simulink model "three_phase_bidirectional_EV_charger_simscape"  (R2019a)
settings: Solver=ode23tb  StartTime=0.0  StopTime=0.2  MaxStep=1e-5  RelTol=1e-5
values from neighbouring files (symbols this model uses):
  C = 33e-6    (= 3.3e-05)    [parameters_for_g2v_closed_loop.m]    (also in parameters_for_v2g_closed_loop.m = 0.002)
  Cf = 300e-3    (= 0.3)    [parameters_for_g2v_closed_loop.m]    (also in parameters_for_v2g_closed_loop.m)
  Co = 2e-3    (= 0.002)    [parameters_for_g2v_closed_loop.m]    (also in parameters_for_v2g_closed_loop.m)
  fline = 50    [parameters_for_g2v_closed_loop.m]    (also in parameters_for_v2g_closed_loop.m)
  fsw_dc = 100e3    (= 100000)    [parameters_for_g2v_closed_loop.m]    (also in parameters_for_v2g_closed_loop.m)
  H = 0.0075    [parameters_for_g2v_closed_loop.m]    (also in parameters_for_v2g_closed_loop.m)
  I = V/R    (= 10)    [parameters_for_g2v_closed_loop.m]    (also in parameters_for_v2g_closed_loop.m = V/(R*(1-D)))
  indicator = 1    [parameters_for_g2v_closed_loop.m]    (also in parameters_for_v2g_closed_loop.m = 0)
  Iqe_max = -Idc_max/K    (= -16.4102564103)    [parameters_for_g2v_closed_loop.m]    (also in parameters_for_v2g_closed_loop.m)
  Kic = Kpc/Tc    (= 4545.45454545)    [parameters_for_g2v_closed_loop.m]    (also in parameters_for_v2g_closed_loop.m)
  Kic_dc = 6749.8    [parameters_for_g2v_closed_loop.m]    (also in parameters_for_v2g_closed_loop.m = 9270.6)
  Kipll = Kpll/Tpll    [parameters_for_g2v_closed_loop.m]    (also in parameters_for_v2g_closed_loop.m)
  Kiv = Kpv/Tv_ac    [parameters_for_g2v_closed_loop.m]    (also in parameters_for_v2g_closed_loop.m)
  Kiv_dc = 15687    [parameters_for_g2v_closed_loop.m]    (also in parameters_for_v2g_closed_loop.m = 1260000)
  Kpc = Kc    (= 32.7272727273)    [parameters_for_g2v_closed_loop.m]    (also in parameters_for_v2g_closed_loop.m)
  Kpc_dc = 0.3    [parameters_for_g2v_closed_loop.m]    (also in parameters_for_v2g_closed_loop.m = 0.29)
  Kpll = (1/Vm)*(1/(alfa_pll*Tsamp_ac))    [parameters_for_g2v_closed_loop.m]    (also in parameters_for_v2g_closed_loop.m)
  Kpv = Kv    [parameters_for_g2v_closed_loop.m]    (also in parameters_for_v2g_closed_loop.m)
  Kpv_dc = 6.9    [parameters_for_g2v_closed_loop.m]    (also in parameters_for_v2g_closed_loop.m = 625.3)
  L = 250e-6    (= 0.00025)    [parameters_for_g2v_closed_loop.m]    (also in parameters_for_v2g_closed_loop.m)
  Lg = 1e-3    (= 0.001)    [parameters_for_g2v_closed_loop.m]    (also in parameters_for_v2g_closed_loop.m)
  Li = 1.6e-3    (= 0.0016)    [parameters_for_g2v_closed_loop.m]    (also in parameters_for_v2g_closed_loop.m)
  Ls = 1e-3    (= 0.001)    [parameters_for_g2v_closed_loop.m]    (also in parameters_for_v2g_closed_loop.m)
  R = V/Iload    (= 50)    [parameters_for_g2v_closed_loop.m]    (also in parameters_for_v2g_closed_loop.m = 1000000)
  Resr = 6e-3    (= 0.006)    [parameters_for_g2v_closed_loop.m]    (also in parameters_for_v2g_closed_loop.m = 0)
  Rf = 0.25    [parameters_for_g2v_closed_loop.m]    (also in parameters_for_v2g_closed_loop.m)
  RL = 10e-3    (= 0.01)    [parameters_for_g2v_closed_loop.m]    (also in parameters_for_v2g_closed_loop.m)
  Rs = 0.5    [parameters_for_g2v_closed_loop.m]    (also in parameters_for_v2g_closed_loop.m)
  T1 = Tsamp_ac/10    (= 5e-06)    [parameters_for_g2v_closed_loop.m]    (also in parameters_for_v2g_closed_loop.m)
  T2 = Tsamp_ac/10    (= 5e-06)    [parameters_for_g2v_closed_loop.m]    (also in parameters_for_v2g_closed_loop.m)
  Tsamp_ac = Tsw_ac/2    (= 5e-05)    [parameters_for_g2v_closed_loop.m]    (also in parameters_for_v2g_closed_loop.m)
  Tsamp_dc = Tsw_dc/2    (= 5e-06)    [parameters_for_g2v_closed_loop.m]    (also in parameters_for_v2g_closed_loop.m)
  V = 500    [parameters_for_g2v_closed_loop.m]    (also in parameters_for_v2g_closed_loop.m = 800)
  Vdc = 800    [parameters_for_g2v_closed_loop.m]    (also in parameters_for_v2g_closed_loop.m)
  Vm = 325    [parameters_for_g2v_closed_loop.m]    (also in parameters_for_v2g_closed_loop.m)
  VM = 4    [parameters_for_g2v_closed_loop.m]    (also in parameters_for_v2g_closed_loop.m)
undefined symbols (not defined in the file or in its folder): Ion, Lithium
libraries: powerlib x58, simulink x9, powerlib_meascontrol x1, electricdrivelib x1
(part 1 of 2)
settings Model: Creator=Görkem  LastModifiedBy=gsahi
settings DataIOCC: ReturnWorkspaceOutputs=off
settings DebuggingCC: ParameterOverflowMsg=none
settings SimscapeCC: SimscapeLogType=all

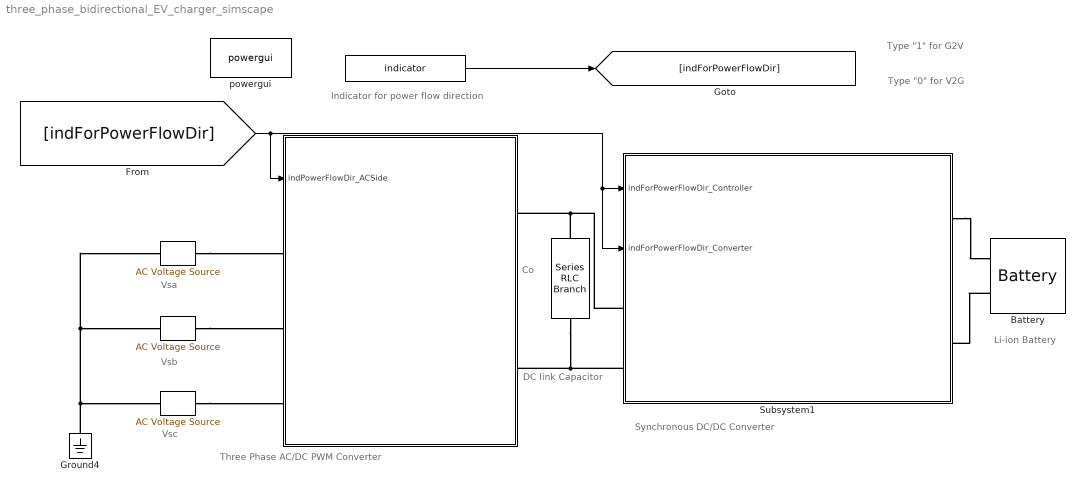
== system three_phase_bidirectional_EV_charger_simscape ==
  note: Vsa
  note: DC link
      | Capacitor
  note: Synchronous DC/DC Converter
  note: Three Phase AC/DC PWM Converter
  note: Indicator for power flow direction
  note: Type "1" for G2V
  note: Type "0" for V2G
  note: Vsb
  note: Vsc
  note: Li-ion
      | Battery
  note: Co
  " " : powerlib/Elements/Series RLC Branch  LConnTagsString=__new0  RConnTagsString=__new0  BranchType=C  Resistance=5  Inductance=1e-3  SetiL0=off  InitialCurrent=0  Capacitance=Co  Setx0=on  InitialVoltage=Vdc  Measurements=None
      settings: SourceProductName=Simscape Electrical
  " " : Constant  Value=indicator
  "  " : powerlib/Electrical Sources/AC Voltage Source  Amplitude=Vm  Phase=0  Frequency=fline  SampleTime=0  Measurements=None  BusType=swing  Pref=10e3  Qref=0  Qmin=-inf  Qmax=+inf
      settings: SourceProductName=Simscape Electrical
  "   " : powerlib/Electrical Sources/AC Voltage Source  Amplitude=Vm  Phase=-120  Frequency=fline  SampleTime=0  Measurements=None  BusType=swing  Pref=10e3  Qref=0  Qmin=-inf  Qmax=+inf
      settings: SourceProductName=Simscape Electrical
  "    " : powerlib/Electrical Sources/AC Voltage Source  Amplitude=Vm  Phase=-240  Frequency=fline  SampleTime=0  Measurements=None  BusType=swing  Pref=10e3  Qref=0  Qmin=-inf  Qmax=+inf
      settings: SourceProductName=Simscape Electrical
  "          " : Subsystem
  Battery : electricdrivelib/Extra Sources/Battery  BatType=Lithium-Ion  ShowTempParam=off  ThermalPreset=no  ShowAgeParam=off  NomV=Vbat_nom  NomQ=BatCap  SOC=SOC_3  Batt_Tr=T_bat  PresetModel=off  MaxQ=30  MinV=215  FullV=530  Dis_rate=13  R=0.14307  Normal_OP=27.1304  expZone="[463.7016      1.473913]"  current=[6.5 13 32.5]  Units=Time  Tci=20  NomT=20  T2=-30  MaxQ2=4.8  FullV2=7.1  Normal_OP2=5.655  expZone2="[6.58           1]"  Rca=0.6  ti=2000  Dp=0  Neq0=0  Tsim=1e6  Ta1=25  Qeol=5.4*0.9  Reol=0.013333*1.2  Char_age=[2.3478, 3]  Dis_age=[2.3478, 10]  N1=1500  N2=10500  N3=1000  N4=1400  Ta2=45  N5=950
      settings: SourceProductName=Simscape Electrical
  Ground4 : powerlib/Elements/Ground  LConnTagsString=a
      settings: SourceProductName=Simscape Electrical
  Subsystem1 : Subsystem
  powergui : powerlib/powergui  Priority=1  SimulationMode=Continuous  SampleTime=Tsamp_ac  frequency=60  Iterations=50  frequencyindice=0  Pbase=100e6  ErrMax=1e-4  UnitsV=kV  UnitsW=MW  buscounter=0  FunctionMessages=off  echomessages=off  EnableUseOfTLC=off  CurrentSourceSwitches=off  DisableSnubberDevices=off  DisableRonSwitches=off  DisableVfSwitches=off  DisplayEquations=off  AutomaticDiscreteSolvers=off  SolverType=Tustin/Backward Euler (TBE)  Interpol=off  ExternalGateDelay=off  methode=off  Ts=100  x0status=blocks  SPID=on  SwTol=0  HookPort=off  NonlinearTolerance=0  nMaxIteration=15  ContinueOnMaxIteration=off  RestoreLinks=warning  ResistiveCurrentMeasurement=off  Frange=[0:2:500]  Ylog=off  Xlog=on  ShowGrid=off  save=off  variable=ZData  structure=I_line  ZoomFFT=off  StartTime=0.04  cycles=1  DisplayStyle=3  fundamental=50  FreqAxis=on  MaxFrequency=1000  frequencyindicesteady=1  RmsSteady=1  display=off
      settings: SourceProductName=Simscape Electrical
  wires:
  " "/1 -> [indForPowerFlowDir]
  [indForPowerFlowDir] -> Subsystem1/1(indForPowerFlowDir_Controller), Subsystem1/2(indForPowerFlowDir_Converter), "          "/1(indPowerFlowDir_ACSide)
  connections:
  "   "/RConn1 -- "          "/LConn2
  "    "/RConn1 -- "          "/LConn3
  " "/LConn1 -- Subsystem1/LConn1 -- "          "/RConn1
  " "/RConn1 -- Subsystem1/LConn2 -- "          "/RConn2
  Battery/LConn2 -- Subsystem1/RConn2
  Subsystem1/RConn1 -- Battery/LConn1
  Ground4/LConn1 -- "  "/LConn1 -- "   "/LConn1 -- "    "/LConn1
  "  "/RConn1 -- "          "/LConn1

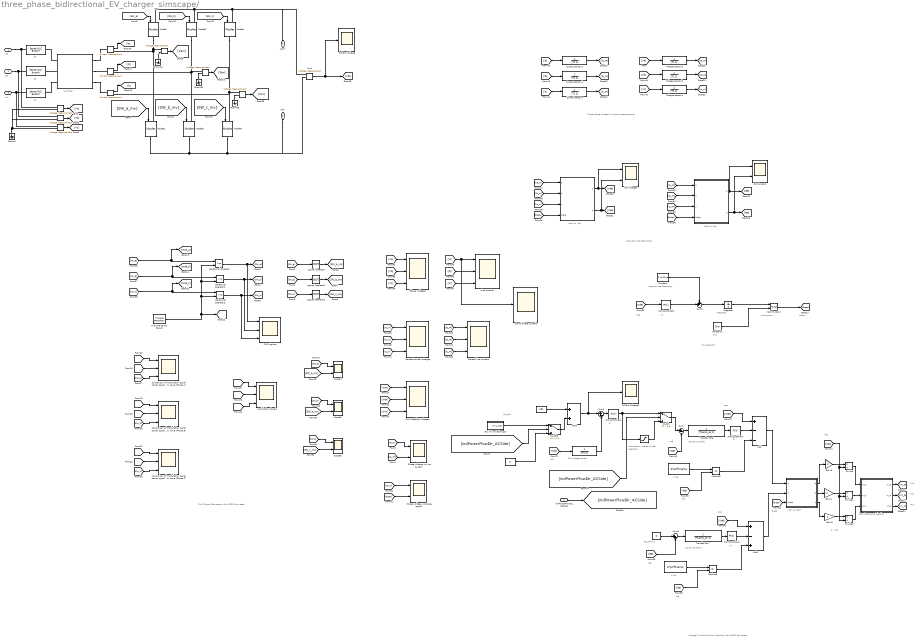
== system three_phase_bidirectional_EV_charger_simscape/           ==
  note: w*Le
  note: "abc" to "dq"
  note: Vsa
  note: Three phase voltage & current measurements
  note: Clark-Park Transformation
  note: PLL algorithm
  note: Vsb
  note: Vsc
  note: Za
  note: Zb
  note: Zc
  note: LCL Filter
  note: Voltage & Current Control Algorithm For AC/DC Converter
  note: PWM Signal Generation For AC/DC Converter
  note: "abc" to "dq"
  note: w*Le
  note: DC voltage sensor
  note: Vdc_ref
  note: Activate for
      | inverter mode
      | operation
  note: Sampling delay
  note: Sampling delay
  note: "dq" to "abc"
  note: Ide_ref = 0
  note: Zero Sequence
      | Injection
  note: Iqe
  note: Ide
  note: Vde
  note: Vqe
  note: Iqe
  note: Ide
  note: PI
  note: PI
  note: Vdc
  note: Vdc
  note: theta
  note: m_a
  note: m_b
  note: m_c
  note: PI
  note: 2 / Vdc
  note: PI
  note: Vde
  note: angular line
      | frequency
  note: integrator
  note: theta
  note: 2*pi
  note: modulation
  indPowerFlowDir_ACSide : Inport
  " " : powerlib/Measurements/Current Measurement  PhasorSimulation=off  OutputType=Complex  PSBequivalent=0
      settings: SourceProductName=Simscape Electrical
  " " : powerlib/Measurements/Current Measurement  PhasorSimulation=off  OutputType=Complex  PSBequivalent=0
      settings: SourceProductName=Simscape Electrical
  " " : powerlib/Measurements/Current Measurement  PhasorSimulation=off  OutputType=Complex  PSBequivalent=0
      settings: SourceProductName=Simscape Electrical
  "     " : powerlib/Elements/Series RLC Branch  LConnTagsString=__new0  RConnTagsString=__new0  BranchType=RL  Resistance=Rs  Inductance=Ls  SetiL0=off  InitialCurrent=0  Capacitance=1e-6  Setx0=off  InitialVoltage=0  Measurements=None
      settings: SourceProductName=Simscape Electrical
  "      " : powerlib/Elements/Series RLC Branch  LConnTagsString=__new0  RConnTagsString=__new0  BranchType=RL  Resistance=Rs  Inductance=Ls  SetiL0=off  InitialCurrent=0  Capacitance=1e-6  Setx0=off  InitialVoltage=0  Measurements=None
      settings: SourceProductName=Simscape Electrical
  "       " : powerlib/Elements/Series RLC Branch  LConnTagsString=__new0  RConnTagsString=__new0  BranchType=RL  Resistance=Rs  Inductance=Ls  SetiL0=off  InitialCurrent=0  Capacitance=1e-6  Setx0=off  InitialVoltage=0  Measurements=None
      settings: SourceProductName=Simscape Electrical
   {,,,} (4 alike) : powerlib/Measurements/Voltage Measurement  PhasorSimulation=off  OutputType=Complex  PSBequivalent=0
      settings: SourceProductName=Simscape Electrical
  "        " : Subsystem
  "            " : Subsystem
  "                    " : Subsystem
  " " : Constant  Value=Vdc
  " " : Constant  Value=0
  " " : Constant  Value=2*pi*fline*Ls
  "                                                " : Constant  Value=2*pi*fline*Ls
  "                                                                                   " : TransferFcn  Denominator=[T1 1]
  "                                                                                                                                                                  " : Saturate  UpperLimit=Iqe_max  LowerLimit=-inf
  "                                                                                                                                                                                                      " : Constant  Value=0
  "                                                                                                                                                                                                                                                   " : Subsystem
  "                                                                                                                                                                                                                                                              " : Subsystem
  "                                                                                                                                                                                                                                                                                             " : powerlib/Measurements/Voltage Measurement  PhasorSimulation=off  OutputType=Complex  PSBequivalent=0
      settings: SourceProductName=Simscape Electrical
  "                                                                                                                                                                                                                                                                                               " : powerlib/Measurements/Voltage Measurement  PhasorSimulation=off  OutputType=Complex  PSBequivalent=0
      settings: SourceProductName=Simscape Electrical
  Add : Sum  Inputs=+--
  Add1 : Sum  Inputs=+-+
  Add2 : Sum
  Constant : Constant  Value=2*pi*fline
  Constant1 : Constant  Value=2*pi
  Current sensor a : TransferFcn  Denominator=[T2 1]
  Current sensor b : TransferFcn  Denominator=[T2 1]
  Current sensor c : TransferFcn  Denominator=[T2 1]
  DC Bus Voltage : Scope
  DC Bus Voltage1 : Scope
  DC link variation g2v : Subsystem
  DQ Currents : Scope  NumInputPorts=2
  DQ Voltages : Scope  NumInputPorts=2
  Divide : Product  Inputs=*/
  Divide1 : Product  Inputs=*/
  Divide2 : Product  Inputs=*/
  Gain3 : Gain  Gain=2
  Gain4 : Gain  Gain=2
  Gain5 : Gain  Gain=2
  Ground{,1..3} (4 alike) : powerlib/Elements/Ground  LConnTagsString=a
      settings: SourceProductName=Simscape Electrical
  Integrator : Integrator
  "Line currents " : Scope  NumInputPorts=3
  Logical Operator : Logic  Operator=NOT  AllPortsSameDT=off  OutDataTypeStr=boolean
  Logical Operator1 : Logic  Operator=NOT  AllPortsSameDT=off  OutDataTypeStr=boolean
  Logical Operator2 : Logic  Operator=NOT  AllPortsSameDT=off  OutDataTypeStr=boolean
  Math Function : Math  Operator=mod  SaturateOnIntegerOverflow=on
  Mosfet{,1..4,6} (6 alike) : powerlib/Power Electronics/Mosfet  Ron=Ron_ac  Lon=0  Rd=0  Vfd=Von_ac  IC=0  Rs=1e5  Cs=inf  Measurements=off
      settings: SourceProductName=Simscape Electrical
  PID Controller1 : simulink/Continuous/PID Controller  Controller=PI  Form=Parallel  TimeDomain=Continuous-time  SampleTime=-1  IntegratorMethod=Forward Euler  FilterMethod=Forward Euler  ControllerParametersSource=internal  P=Kpc  I=Kic  D=0  UseFilter=on  N=100  TunerSelectOption=Transfer Function Based (PID Tuner App)  InitialConditionSource=internal  InitialConditionForIntegrator=0  InitialConditionForFilter=0  DifferentiatorICPrevScaledInput=0  ExternalReset=none  TrackingMode=off  Kt=1  LimitOutput=on  UpperSaturationLimit=Vdc/2  LowerSaturationLimit=-Vdc/2  LinearizeAsGain=on  AntiWindupMode=clamping  Kb=1  POutMin=[]  POutMax=[]  IOutMin=[]  IOutMax=[]  DOutMin=[]  DOutMax=[]  NOutMin=[]  NOutMax=[]  SumOutMin=[]  SumOutMax=[]  SaturationOutMin=[]  SaturationOutMax=[]  PParamMin=[]  PParamMax=[]  IParamMin=[]  IParamMax=[]  DParamMin=[]  DParamMax=[]  NParamMin=[]  NParamMax=[]  KbParamMin=[]  KbParamMax=[]  KtParamMin=[]  KtParamMax=[]  KbOutMin=[]  KbOutMax=[]  KtOutMin=[]  KtOutMax=[]  IntegratorOutMin=[]  IntegratorOutMax=[]  FilterOutMin=[]  FilterOutMax=[]  SumI1OutMin=[]  SumI1OutMax=[]  SumI2OutMin=[]  SumI2OutMax=[]  SumI3OutMin=[]  SumI3OutMax=[]  SumI4OutMin=[]  SumI4OutMax=[]  SumDOutMin=[]  SumDOutMax=[]  DifferentiatorOutMin=[]  DifferentiatorOutMax=[]  FilterDiffOutCoefMin=[]  FilterDiffOutCoefMax=[]  ReciprocalOutMin=[]  ReciprocalOutMax=[]  SumDenOutMin=[]  SumDenOutMax=[]  SumNumOutMin=[]  SumNumOutMax=[]  DivideOutMin=[]  DivideOutMax=[]  IntegratorContinuousStateAttributes=''  IntegratorStateMustResolveToSignalObject=off  IntegratorRTWStateStorageClass=Auto  FilterContinuousStateAttributes=''  FilterStateMustResolveToSignalObject=off  FilterRTWStateStorageClass=Auto  ParallelPVariant=InternalParameters  IdealPVariant=Disabled  IVariant=InternalParameters  DVariant=Disabled  IntegratorVariant=Continuous  SatVariant=Enabled  AWVariant=ContClampingParallel  PCopyVariant=Disabled  TRVariant=Disabled  FdbkBlocksVariant=Forward  IdealPFdbkVariant=Disabled  SatFdbkVariant=Disabled  DerivativeFilterVariant=Disabled  NVariant=Disabled  NCopyVariant=Disabled_SignalSpec  FilterICVariant=Disabled  IntegratorICVariant=InternalICs  ExternalResetVariant=Disabled  TRSumVariant=Passthrough  SumFdbkVariant=Disabled  SumVariant=Sum_PI
  PID Controller2 : simulink/Continuous/PID Controller  Controller=PI  Form=Parallel  TimeDomain=Continuous-time  SampleTime=-1  IntegratorMethod=Forward Euler  FilterMethod=Forward Euler  ControllerParametersSource=internal  P=Kpv  I=Kiv  D=0  UseFilter=on  N=100  TunerSelectOption=Transfer Function Based (PID Tuner App)  InitialConditionSource=internal  InitialConditionForIntegrator=0  InitialConditionForFilter=0  DifferentiatorICPrevScaledInput=0  ExternalReset=none  TrackingMode=off  Kt=1  LimitOutput=off  UpperSaturationLimit=200  LowerSaturationLimit=-200  LinearizeAsGain=on  AntiWindupMode=clamping  Kb=1  POutMin=[]  POutMax=[]  IOutMin=[]  IOutMax=[]  DOutMin=[]  DOutMax=[]  NOutMin=[]  NOutMax=[]  SumOutMin=[]  SumOutMax=[]  SaturationOutMin=[]  SaturationOutMax=[]  PParamMin=[]  PParamMax=[]  IParamMin=[]  IParamMax=[]  DParamMin=[]  DParamMax=[]  NParamMin=[]  NParamMax=[]  KbParamMin=[]  KbParamMax=[]  KtParamMin=[]  KtParamMax=[]  KbOutMin=[]  KbOutMax=[]  KtOutMin=[]  KtOutMax=[]  IntegratorOutMin=[]  IntegratorOutMax=[]  FilterOutMin=[]  FilterOutMax=[]  SumI1OutMin=[]  SumI1OutMax=[]  SumI2OutMin=[]  SumI2OutMax=[]  SumI3OutMin=[]  SumI3OutMax=[]  SumI4OutMin=[]  SumI4OutMax=[]  SumDOutMin=[]  SumDOutMax=[]  DifferentiatorOutMin=[]  DifferentiatorOutMax=[]  FilterDiffOutCoefMin=[]  FilterDiffOutCoefMax=[]  ReciprocalOutMin=[]  ReciprocalOutMax=[]  SumDenOutMin=[]  SumDenOutMax=[]  SumNumOutMin=[]  SumNumOutMax=[]  DivideOutMin=[]  DivideOutMax=[]  IntegratorContinuousStateAttributes=''  IntegratorStateMustResolveToSignalObject=off  IntegratorRTWStateStorageClass=Auto  FilterContinuousStateAttributes=''  FilterStateMustResolveToSignalObject=off  FilterRTWStateStorageClass=Auto  ParallelPVariant=InternalParameters  IdealPVariant=Disabled  IVariant=InternalParameters  DVariant=Disabled  IntegratorVariant=Continuous  SatVariant=Disabled  AWVariant=Passthrough  PCopyVariant=Disabled  TRVariant=Disabled  FdbkBlocksVariant=Forward  IdealPFdbkVariant=Disabled  SatFdbkVariant=Disabled  DerivativeFilterVariant=Disabled  NVariant=Disabled  NCopyVariant=Disabled_SignalSpec  FilterICVariant=Disabled  IntegratorICVariant=InternalICs  ExternalResetVariant=Disabled  TRSumVariant=Passthrough  SumFdbkVariant=Disabled  SumVariant=Sum_PI
  PID Controller3 : simulink/Continuous/PID Controller  Controller=PI  Form=Parallel  TimeDomain=Continuous-time  SampleTime=-1  IntegratorMethod=Forward Euler  FilterMethod=Forward Euler  ControllerParametersSource=internal  P=Kpll  I=Kipll  D=0  UseFilter=on  N=100  TunerSelectOption=Transfer Function Based (PID Tuner App)  InitialConditionSource=internal  InitialConditionForIntegrator=0  InitialConditionForFilter=0  DifferentiatorICPrevScaledInput=0  ExternalReset=none  TrackingMode=off  Kt=1  LimitOutput=off  UpperSaturationLimit=inf  LowerSaturationLimit=-inf  LinearizeAsGain=on  AntiWindupMode=none  Kb=1  POutMin=[]  POutMax=[]  IOutMin=[]  IOutMax=[]  DOutMin=[]  DOutMax=[]  NOutMin=[]  NOutMax=[]  SumOutMin=[]  SumOutMax=[]  SaturationOutMin=[]  SaturationOutMax=[]  PParamMin=[]  PParamMax=[]  IParamMin=[]  IParamMax=[]  DParamMin=[]  DParamMax=[]  NParamMin=[]  NParamMax=[]  KbParamMin=[]  KbParamMax=[]  KtParamMin=[]  KtParamMax=[]  KbOutMin=[]  KbOutMax=[]  KtOutMin=[]  KtOutMax=[]  IntegratorOutMin=[]  IntegratorOutMax=[]  FilterOutMin=[]  FilterOutMax=[]  SumI1OutMin=[]  SumI1OutMax=[]  SumI2OutMin=[]  SumI2OutMax=[]  SumI3OutMin=[]  SumI3OutMax=[]  SumI4OutMin=[]  SumI4OutMax=[]  SumDOutMin=[]  SumDOutMax=[]  DifferentiatorOutMin=[]  DifferentiatorOutMax=[]  FilterDiffOutCoefMin=[]  FilterDiffOutCoefMax=[]  ReciprocalOutMin=[]  ReciprocalOutMax=[]  SumDenOutMin=[]  SumDenOutMax=[]  SumNumOutMin=[]  SumNumOutMax=[]  DivideOutMin=[]  DivideOutMax=[]  IntegratorContinuousStateAttributes=''  IntegratorStateMustResolveToSignalObject=off  IntegratorRTWStateStorageClass=Auto  FilterContinuousStateAttributes=''  FilterStateMustResolveToSignalObject=off  FilterRTWStateStorageClass=Auto  ParallelPVariant=InternalParameters  IdealPVariant=Disabled  IVariant=InternalParameters  DVariant=Disabled  IntegratorVariant=Continuous  SatVariant=Disabled  AWVariant=Passthrough  PCopyVariant=Disabled  TRVariant=Disabled  FdbkBlocksVariant=Forward  IdealPFdbkVariant=Disabled  SatFdbkVariant=Disabled  DerivativeFilterVariant=Disabled  NVariant=Disabled  NCopyVariant=Disabled_SignalSpec  FilterICVariant=Disabled  IntegratorICVariant=InternalICs  ExternalResetVariant=Disabled  TRSumVariant=Passthrough  SumFdbkVariant=Disabled  SumVariant=Sum_PI
  PID Controller4 : simulink/Continuous/PID Controller  Controller=PI  Form=Parallel  TimeDomain=Continuous-time  SampleTime=-1  IntegratorMethod=Forward Euler  FilterMethod=Forward Euler  ControllerParametersSource=internal  P=Kpc  I=Kic  D=0  UseFilter=on  N=100  TunerSelectOption=Transfer Function Based (PID Tuner App)  InitialConditionSource=internal  InitialConditionForIntegrator=0  InitialConditionForFilter=0  DifferentiatorICPrevScaledInput=0  ExternalReset=none  TrackingMode=off  Kt=1  LimitOutput=on  UpperSaturationLimit=Vdc/2  LowerSaturationLimit=-Vdc/2  LinearizeAsGain=on  AntiWindupMode=clamping  Kb=1  POutMin=[]  POutMax=[]  IOutMin=[]  IOutMax=[]  DOutMin=[]  DOutMax=[]  NOutMin=[]  NOutMax=[]  SumOutMin=[]  SumOutMax=[]  SaturationOutMin=[]  SaturationOutMax=[]  PParamMin=[]  PParamMax=[]  IParamMin=[]  IParamMax=[]  DParamMin=[]  DParamMax=[]  NParamMin=[]  NParamMax=[]  KbParamMin=[]  KbParamMax=[]  KtParamMin=[]  KtParamMax=[]  KbOutMin=[]  KbOutMax=[]  KtOutMin=[]  KtOutMax=[]  IntegratorOutMin=[]  IntegratorOutMax=[]  FilterOutMin=[]  FilterOutMax=[]  SumI1OutMin=[]  SumI1OutMax=[]  SumI2OutMin=[]  SumI2OutMax=[]  SumI3OutMin=[]  SumI3OutMax=[]  SumI4OutMin=[]  SumI4OutMax=[]  SumDOutMin=[]  SumDOutMax=[]  DifferentiatorOutMin=[]  DifferentiatorOutMax=[]  FilterDiffOutCoefMin=[]  FilterDiffOutCoefMax=[]  ReciprocalOutMin=[]  ReciprocalOutMax=[]  SumDenOutMin=[]  SumDenOutMax=[]  SumNumOutMin=[]  SumNumOutMax=[]  DivideOutMin=[]  DivideOutMax=[]  IntegratorContinuousStateAttributes=''  IntegratorStateMustResolveToSignalObject=off  IntegratorRTWStateStorageClass=Auto  FilterContinuousStateAttributes=''  FilterStateMustResolveToSignalObject=off  FilterRTWStateStorageClass=Auto  ParallelPVariant=InternalParameters  IdealPVariant=Disabled  IVariant=InternalParameters  DVariant=Disabled  IntegratorVariant=Continuous  SatVariant=Enabled  AWVariant=ContClampingParallel  PCopyVariant=Disabled  TRVariant=Disabled  FdbkBlocksVariant=Forward  IdealPFdbkVariant=Disabled  SatFdbkVariant=Disabled  DerivativeFilterVariant=Disabled  NVariant=Disabled  NCopyVariant=Disabled_SignalSpec  FilterICVariant=Disabled  IntegratorICVariant=InternalICs  ExternalResetVariant=Disabled  TRSumVariant=Passthrough  SumFdbkVariant=Disabled  SumVariant=Sum_PI
  PWM Rectifier Voltages : Scope  NumInputPorts=3
  PWM signals : Scope  NumInputPorts=3
  Phase voltage vs line current : Scope  NumInputPorts=2
  Phase voltage vs phase angle : Scope  NumInputPorts=2
  Phase voltages : Scope  NumInputPorts=3
  Product2 : Product
  Product3 : Product
  Relational Operator : RelationalOperator  OutDataTypeStr=boolean  RndMeth=Simplest
  Relational Operator1 : RelationalOperator  OutDataTypeStr=boolean  RndMeth=Simplest
  Relational Operator2 : RelationalOperator  OutDataTypeStr=boolean  RndMeth=Simplest
  Scope4 : Scope  NumInputPorts=2
  Scope5 : Scope  NumInputPorts=2
  Scope6 : Scope  NumInputPorts=2
  Sensed line currents : Scope  NumInputPorts=3
  Sensed source voltages : Scope  NumInputPorts=3
  Sum1 : Sum  Inputs=|+-
  Sum6 : Sum  Inputs=++|
  Sum7 : Sum  Inputs=|+-
  Sum8 : Sum  Inputs=|+-
  Switch : Switch  Criteria=u2 > Threshold  Threshold=0.5
  Switch3 : Switch  Criteria=u2 > Threshold  Threshold=0.5
  Transfer Fcn6 : TransferFcn  Denominator=[Tsamp_ac 1]
  Transfer Fcn7 : TransferFcn  Denominator=[Tsamp_ac 1]
  Triangle Carrier Signal : powerlib_meascontrol/Pulse & Signal Generators/Triangle Generator  Freq=fsw_ac  Phase=-90  Ts=0
      settings: SourceProductName=Simscape Electrical
  Voltage sensor a : TransferFcn  Denominator=[T1 1]
  Voltage sensor b : TransferFcn  Denominator=[T1 1]
  Voltage sensor c : TransferFcn  Denominator=[T1 1]
  Vout : powerlib/Measurements/Voltage Measurement  PhasorSimulation=off  OutputType=Complex  PSBequivalent=0
      settings: SourceProductName=Simscape Electrical
  comparison of modulation signal carrier signal and pwm wave (Phase A) : Scope  NumInputPorts=3
  comparison of modulation signal carrier signal and pwm wave (Phase B) : Scope  NumInputPorts=3
  comparison of modulation signal carrier signal and pwm wave (Phase C) : Scope  NumInputPorts=3
  modulation signals : Scope  NumInputPorts=3
  one of phase currents : Scope
  " " : PMIOPort  Side=Left
  "  " : PMIOPort  Port=2  Side=Left
  "   " : PMIOPort  Port=3  Side=Left
  Vdc+ : PMIOPort  Port=4  Side=Right
  Vdc- : PMIOPort  Port=5  Side=Right
  wires:
  " "/1 -> [Va]
  Vout/1 -> [Vdc], DC Bus Voltage/1
  " "/1 -> [Vb]
  [SW_c] -> Mosfet1/1
  " "/1 -> [Ia]
  " "/1 -> [Ib]
  "                                                                                                                                                                                                                                                                                               "/1 -> [Vbn]
  [SW_c_inv] -> Mosfet4/1
  " "/1 -> [Ic]
  "                                                                                                                                                                                                                                                                                             "/1 -> [Van]
  [SW_b] -> Mosfet6/1
  [SW_a] -> Mosfet/1
  " "/1 -> [Vcn]
  " "/1 -> [Vc]
  [SW_a_inv] -> Mosfet2/1
  [SW_b_inv] -> Mosfet3/1
  Sum1/1 -> PID Controller2/1
  "                                                                                                                                                                  "/1 -> Switch/3
  [theta] -> "                    "/4(theta)
  [Ib] -> Current sensor b/1
  Sum6/1 -> Integrator/1
  [theta] -> Phase voltage vs phase angle/2
  [Iqe] -> Product3/2
  [Vb_m] -> Sensed source voltages/2
  Current sensor c/1 -> [Ic_m]
  Gain4/1 -> Divide1/1
  "                                                                                                                                                                                                                                                   "/3(c) -> Gain5/1
  [Vb] -> Phase voltages/2
  [Vde] -> PID Controller3/1
  Integrator/1 -> Math Function/1
  Sum8/1 -> Transfer Fcn7/1
  [Vde] -> Add1/1
  [Vb] -> Voltage sensor b/1
  [Ib] -> "Line currents "/2
  [Va_m] -> Sensed source voltages/1
  [Vqe] -> Add/1
  [Ic] -> "Line currents "/3
  [SW_b_inv] -> Scope5/2
  Add1/1 -> "                                                                                                                                                                                                                                                   "/2(d)
  Constant1/1 -> Math Function/2
  [SW_a] -> Scope4/1
  [Vc] -> Voltage sensor c/1
  Math Function/1 -> [theta]
  [mod_a] -> comparison of modulation signal carrier signal and pwm wave (Phase A)/1
  PID Controller1/1 -> Add1/2
  [Vc_m] -> "            "/3(c)
  Transfer Fcn7/1 -> PID Controller1/1
  Product3/1 -> Add1/3
  Transfer Fcn6/1 -> PID Controller4/1
  PID Controller3/1 -> Sum6/2
  [Vb_m] -> "            "/2(b)
  [carrier] -> comparison of modulation signal carrier signal and pwm wave (Phase A)/2
  Constant/1 -> Sum6/1
  [Ic_m] -> "                    "/3(c)
  [Ia] -> Current sensor a/1
  "                    "/2(q) -> DQ Currents/2, [Iqe]
  [SW_b] -> comparison of modulation signal carrier signal and pwm wave (Phase B)/3
  Add/1 -> "                                                                                                                                                                                                                                                   "/1(q)
  Current sensor b/1 -> [Ib_m]
  [Ic] -> Current sensor c/1
  Voltage sensor b/1 -> [Vb_m]
  [Va] -> Voltage sensor a/1
  [mod_c] -> comparison of modulation signal carrier signal and pwm wave (Phase C)/1
  "            "/2(q) -> DQ Voltages/2, [Vqe]
  [SW_c_inv] -> Scope6/2
  [Va_m] -> Phase voltage vs phase angle/1
  [SW_a_inv] -> Scope4/2
  [Ia_m] -> "                    "/1(a)
  "            "/1(d) -> DQ Voltages/1, [Vde]
  [Ia_m] -> Sensed line currents/1
  [SW_a] -> Logical Operator/1
  [Va_m] -> Phase voltage vs line current/1
  [theta] -> "            "/4(theta)
  [Ib_m] -> Sensed line currents/2
  [Ib_m] -> "                    "/2(b)
  [Vcn] -> PWM Rectifier Voltages/3
  [mod_c] -> modulation signals/3
  [mod_a] -> modulation signals/1
  [SW_a] -> comparison of modulation signal carrier signal and pwm wave (Phase A)/3
  [carrier] -> comparison of modulation signal carrier signal and pwm wave (Phase C)/2
  [mod_b] -> modulation signals/2
  Relational Operator1/1 -> PWM signals/2, [SW_b]
  [carrier] -> comparison of modulation signal carrier signal and pwm wave (Phase B)/2
  [SW_b] -> Scope5/1
  [m_a] -> Relational Operator/1, [mod_a]
  [SW_c] -> Scope6/1
  Logical Operator/1 -> [SW_a_inv]
  Logical Operator1/1 -> [SW_b_inv]
  Relational Operator2/1 -> PWM signals/3, [SW_c]
  [SW_b] -> Logical Operator1/1
  [Van] -> PWM Rectifier Voltages/1
  [Vbn] -> PWM Rectifier Voltages/2
  Logical Operator2/1 -> [SW_c_inv]
  Product2/1 -> Add/3
  [Va] -> Phase voltages/1
  "                                                "/1 -> Product2/1
  [Va_m] -> "            "/1(a)
  [Iqe] -> Sum7/2
  PID Controller2/1 -> "                                                                                                                                                                  "/1, Switch/1
  "                                                                                                                                                                                                                                                   "/2(b) -> Gain4/1
  [Ide] -> Product2/2
  Divide/1 -> "                                                                                                                                                                                                                                                              "/1(m_a)
  Gain5/1 -> Divide2/1
  " "/1 -> Product3/1
  Gain3/1 -> Divide/1
  [SW_c] -> Logical Operator2/1
  Switch/1 -> Sum7/1
  [mod_b] -> comparison of modulation signal carrier signal and pwm wave (Phase B)/1
  Voltage sensor a/1 -> [Va_m]
  Relational Operator/1 -> PWM signals/1, [SW_a]
  Divide1/1 -> "                                                                                                                                                                                                                                                              "/2(m_b)
  Triangle Carrier Signal/1 -> [carrier], Relational Operator2/2, Relational Operator1/2, Relational Operator/2
  [Ia_m] -> Phase voltage vs line current/2
  "                                                                                                                                                                                                      "/1 -> Sum8/1
  [Ide] -> Sum8/2
  "                                                                                                                                                                                                                                                   "/1(a) -> Gain3/1
  PID Controller4/1 -> Add/2
  Voltage sensor c/1 -> [Vc_m]
  [m_c] -> Relational Operator2/1, [mod_c]
  [SW_c] -> comparison of modulation signal carrier signal and pwm wave (Phase C)/3
  [Vc] -> Phase voltages/3
  [Ic_m] -> Sensed line currents/3
  [theta] -> "                                                                                                                                                                                                                                                   "/3(theta)
  Sum7/1 -> Transfer Fcn6/1
  "                    "/1(d) -> DQ Currents/1, [Ide]
  [Vdc] -> Divide/2, Divide1/2, Divide2/2
  Divide2/1 -> "                                                                                                                                                                                                                                                              "/3(m_c)
  Current sensor a/1 -> [Ia_m]
  [m_b] -> Relational Operator1/1, [mod_b]
  [Ia] -> one of phase currents/1, "Line currents "/1
  [Vc_m] -> Sensed source voltages/3
  [indPowerFlowDir_ACSide] -> Switch/2
  [Vdc] -> "                                                                                   "/1
  "                                                                                   "/1 -> Sum1/2
  "                                                                                                                                                                                                                                                              "/2(m_b') -> [m_b]
  "                                                                                                                                                                                                                                                              "/3(m_c') -> [m_c]
  "                                                                                                                                                                                                                                                              "/1(m_a') -> [m_a]
  indPowerFlowDir_ACSide/1 -> [indPowerFlowDir_ACSide]
  Add2/1 -> DC Bus Voltage1/1, Sum1/1
  " "/1 -> Add2/1
  DC link variation g2v/1(Vbus_step) -> Switch3/1
  " "/1 -> Switch3/3
  Switch3/1 -> Add2/2
  [indPowerFlowDir_ACSide] -> Switch3/2
  connections:
  Ground1/LConn1 -- "                                                                                                                                                                                                                                                                                             "/LConn2
  Mosfet/RConn1 -- "                                                                                                                                                                                                                                                                                             "/LConn1 -- Mosfet2/LConn1 -- " "/RConn1
  Mosfet3/RConn1 -- Vdc-/RConn1 -- Vout/LConn2 -- Mosfet4/RConn1 -- Mosfet2/RConn1
  Ground/LConn1 -- " "/LConn2
  " "/LConn1 -- " "/RConn1 -- "     "/LConn1
  " "/LConn1 -- "  "/RConn1 -- "      "/LConn1
  "                                                                                                                                                                                                                                                                                               "/LConn1 -- Mosfet6/RConn1 -- Mosfet3/LConn1 -- " "/RConn1
  " "/LConn1 -- "   "/RConn1 -- "       "/LConn1
  Mosfet4/LConn1 -- " "/RConn1 -- Mosfet1/RConn1 -- " "/LConn1
  Ground3/LConn1 -- " "/LConn2
  "                                                                                                                                                                                                                                                                                               "/LConn2 -- Ground2/LConn1
  Mosfet/LConn1 -- Mosfet6/LConn1 -- Vdc+/RConn1 -- Vout/LConn1 -- Mosfet1/LConn1
  "        "/LConn2 -- "      "/RConn1
  "        "/RConn2 -- " "/LConn1
  "        "/LConn1 -- "     "/RConn1
  "        "/LConn3 -- "       "/RConn1
  "        "/RConn1 -- " "/LConn1
  "        "/RConn3 -- " "/LConn1

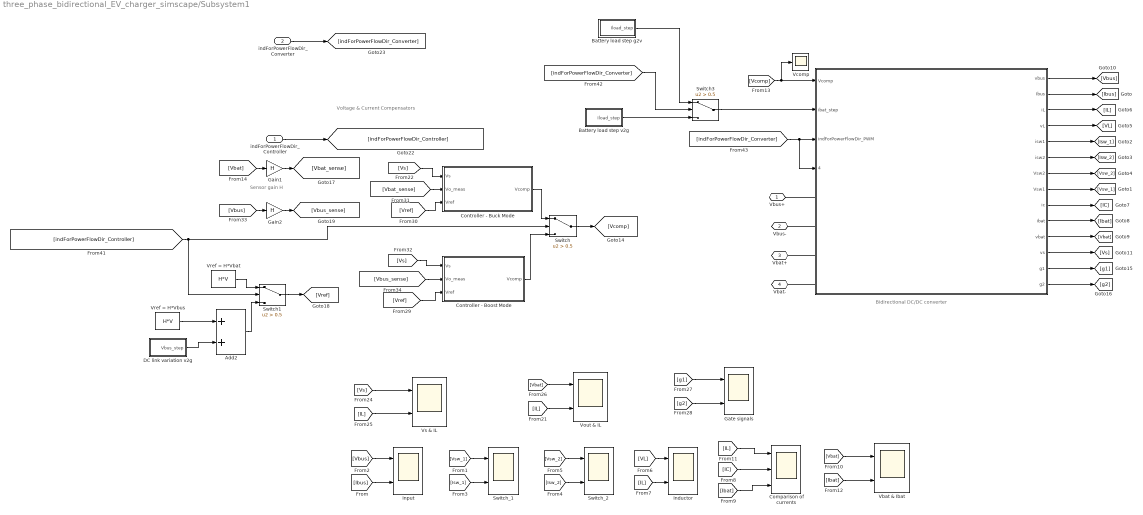
== system three_phase_bidirectional_EV_charger_simscape/Subsystem1 ==
  note: Voltage & Current Compensators
  note: Bidirectional DC/DC converter
  note: Sensor gain
      | H
  indForPowerFlowDir_Controller : Inport
  indForPowerFlowDir_Converter : Inport  Port=2
  "   " : Subsystem
  Add2 : Sum
  Battery load step g2v : Subsystem
  Battery load step v2g : Subsystem
  Comparison of currents : Scope  NumInputPorts=3
  Controller - Boost Mode : Subsystem
  Controller - Buck Mode : Subsystem
  DC link variation v2g : Subsystem
  Gain1 : Gain  Gain=H
  Gain2 : Gain  Gain=H
  Gate signals : Scope  NumInputPorts=2
  Inductor : Scope  NumInputPorts=2
  Input : Scope  NumInputPorts=2
  Switch : Switch  Criteria=u2 > Threshold  Threshold=0.5
  Switch1 : Switch  Criteria=u2 > Threshold  Threshold=0.5
  Switch3 : Switch  Criteria=u2 > Threshold  Threshold=0.5
  Switch_1 : Scope  NumInputPorts=2
  Switch_2 : Scope  NumInputPorts=2
  Vbat & Ibat : Scope  NumInputPorts=2
  Vcomp : Scope
  Vout & IL : Scope  NumInputPorts=2
  Vref = H*Vbat : Constant  Value=H*V
  Vref = H*Vbus : Constant  Value=H*V
  Vs & IL : Scope  NumInputPorts=2
  Vbus+ : PMIOPort  Side=Left
  Vbus- : PMIOPort  Port=2  Side=Left
  Vbat+ : PMIOPort  Port=3  Side=Right
  Vbat- : PMIOPort  Port=4  Side=Right
  wires:
  [Vbus] -> Input/1
  [IL] -> Inductor/2
  "   "/5(isw1) -> [Isw_1]
  [Ibat] -> Comparison of currents/3
  [Vbat] -> Vout & IL/1
  "   "/8(Vsw1) -> [Vsw_1]
  [g2] -> Gate signals/2
  "   "/11(vbat) -> [Vbat]
  [Isw_1] -> Switch_1/2
  "   "/2(Ibus) -> [Ibus]
  [IC] -> Comparison of currents/2
  [Vbus_sense] -> Controller - Boost Mode/2(Vo_meas)
  Gain1/1 -> [Vbat_sense]
  [Vs] -> Controller - Buck Mode/1(Vs)
  [VL] -> Inductor/1
  "   "/9(ic) -> [IC]
  [Vbat] -> Vbat & Ibat/1
  [Ibus] -> Input/2
  [IL] -> Vs & IL/2
  [g1] -> Gate signals/1
  [Vs] -> Controller - Boost Mode/1(Vs)
  [Ibat] -> Vbat & Ibat/2
  [Vs] -> Vs & IL/1
  [Vbat_sense] -> Controller - Buck Mode/2(Vo_meas)
  "   "/14(g2) -> [g2]
  [Vref] -> Controller - Boost Mode/3(Vref)
  [Vbat] -> Gain1/1
  "   "/13(g1) -> [g1]
  [Vref] -> Controller - Buck Mode/3(Vref)
  "   "/10(ibat) -> [Ibat]
  "   "/3(iL) -> [IL]
  "   "/12(vs) -> [Vs]
  [Vcomp] -> "   "/1(Vcomp), Vcomp/1
  [IL] -> Comparison of currents/1
  [Isw_2] -> Switch_2/2
  [Vsw_1] -> Switch_1/1
  [Vsw_2] -> Switch_2/1
  [IL] -> Vout & IL/2
  "   "/7(Vsw2) -> [Vsw_2]
  "   "/6(isw2) -> [Isw_2]
  "   "/1(vbus) -> [Vbus]
  "   "/4(vL) -> [VL]
  [Vbus] -> Gain2/1
  Gain2/1 -> [Vbus_sense]
  [indForPowerFlowDir_Converter] -> "   "/4(" "), "   "/3(indForPowerFlowDir_PWM)
  Controller - Boost Mode/1("Vcomp ") -> Switch/3
  Controller - Buck Mode/1("Vcomp ") -> Switch/1
  [indForPowerFlowDir_Controller] -> Switch/2, Switch1/2
  Switch/1 -> [Vcomp]
  indForPowerFlowDir_Controller/1 -> [indForPowerFlowDir_Controller]
  indForPowerFlowDir_Converter/1 -> [indForPowerFlowDir_Converter]
  Switch3/1 -> "   "/2(ibat_step)
  Battery load step g2v/1(Iload_step) -> Switch3/1
  Battery load step v2g/1(Iload_step) -> Switch3/3
  [indForPowerFlowDir_Converter] -> Switch3/2
  Switch1/1 -> [Vref]
  Vref = H*Vbat/1 -> Switch1/1
  Vref = H*Vbus/1 -> Add2/1
  Add2/1 -> Switch1/3
  DC link variation v2g/1(Vbus_step) -> Add2/2
  connections:
  "   "/LConn1 -- Vbus+/RConn1
  "   "/LConn4 -- Vbat-/RConn1
  "   "/LConn3 -- Vbat+/RConn1
  "   "/LConn2 -- Vbus-/RConn1

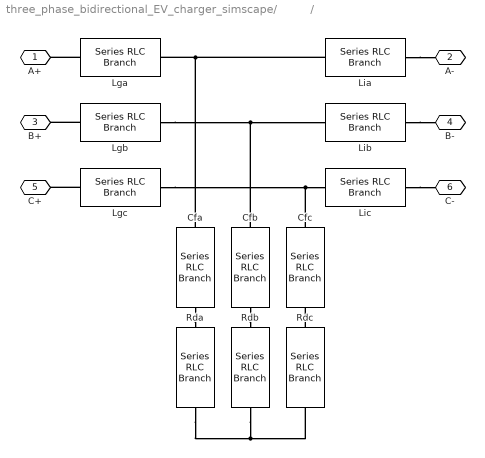
== system three_phase_bidirectional_EV_charger_simscape/          /         ==
  " Rdb" : powerlib/Elements/Series RLC Branch  LConnTagsString=__new0  RConnTagsString=__new0  BranchType=R  Resistance=0.5  Inductance=Ls  SetiL0=off  InitialCurrent=0  Capacitance=Cf  Setx0=off  InitialVoltage=0  Measurements=None
      settings: SourceProductName=Simscape Electrical
  Cfa : powerlib/Elements/Series RLC Branch  LConnTagsString=__new0  RConnTagsString=__new0  BranchType=C  Resistance=Rs  Inductance=Ls  SetiL0=off  InitialCurrent=0  Capacitance=Cf  Setx0=off  InitialVoltage=0  Measurements=None
      settings: SourceProductName=Simscape Electrical
  Cfb : powerlib/Elements/Series RLC Branch  LConnTagsString=__new0  RConnTagsString=__new0  BranchType=C  Resistance=Rs  Inductance=Ls  SetiL0=off  InitialCurrent=0  Capacitance=Cf  Setx0=off  InitialVoltage=0  Measurements=None
      settings: SourceProductName=Simscape Electrical
  Cfc : powerlib/Elements/Series RLC Branch  LConnTagsString=__new0  RConnTagsString=__new0  BranchType=C  Resistance=Rs  Inductance=Ls  SetiL0=off  InitialCurrent=0  Capacitance=Cf  Setx0=off  InitialVoltage=0  Measurements=None
      settings: SourceProductName=Simscape Electrical
  Lga : powerlib/Elements/Series RLC Branch  LConnTagsString=__new0  RConnTagsString=__new0  BranchType=L  Resistance=Rs  Inductance=Lg  SetiL0=off  InitialCurrent=0  Capacitance=1e-6  Setx0=off  InitialVoltage=0  Measurements=None
      settings: SourceProductName=Simscape Electrical
  Lgb : powerlib/Elements/Series RLC Branch  LConnTagsString=__new0  RConnTagsString=__new0  BranchType=L  Resistance=Rs  Inductance=Lg  SetiL0=off  InitialCurrent=0  Capacitance=1e-6  Setx0=off  InitialVoltage=0  Measurements=None
      settings: SourceProductName=Simscape Electrical
  Lgc : powerlib/Elements/Series RLC Branch  LConnTagsString=__new0  RConnTagsString=__new0  BranchType=L  Resistance=Rs  Inductance=Lg  SetiL0=off  InitialCurrent=0  Capacitance=1e-6  Setx0=off  InitialVoltage=0  Measurements=None
      settings: SourceProductName=Simscape Electrical
  Lia : powerlib/Elements/Series RLC Branch  LConnTagsString=__new0  RConnTagsString=__new0  BranchType=L  Resistance=Rs  Inductance=Li  SetiL0=off  InitialCurrent=0  Capacitance=1e-6  Setx0=off  InitialVoltage=0  Measurements=None
      settings: SourceProductName=Simscape Electrical
  Lib : powerlib/Elements/Series RLC Branch  LConnTagsString=__new0  RConnTagsString=__new0  BranchType=L  Resistance=Rs  Inductance=Li  SetiL0=off  InitialCurrent=0  Capacitance=1e-6  Setx0=off  InitialVoltage=0  Measurements=None
      settings: SourceProductName=Simscape Electrical
  Lic : powerlib/Elements/Series RLC Branch  LConnTagsString=__new0  RConnTagsString=__new0  BranchType=L  Resistance=Rs  Inductance=Li  SetiL0=off  InitialCurrent=0  Capacitance=1e-6  Setx0=off  InitialVoltage=0  Measurements=None
      settings: SourceProductName=Simscape Electrical
  Rda : powerlib/Elements/Series RLC Branch  LConnTagsString=__new0  RConnTagsString=__new0  BranchType=R  Resistance=0.5  Inductance=Ls  SetiL0=off  InitialCurrent=0  Capacitance=Cf  Setx0=off  InitialVoltage=0  Measurements=None
      settings: SourceProductName=Simscape Electrical
  Rdc : powerlib/Elements/Series RLC Branch  LConnTagsString=__new0  RConnTagsString=__new0  BranchType=R  Resistance=0.5  Inductance=Ls  SetiL0=off  InitialCurrent=0  Capacitance=Cf  Setx0=off  InitialVoltage=0  Measurements=None
      settings: SourceProductName=Simscape Electrical
  A+ : PMIOPort  Side=Left
  A- : PMIOPort  Port=2  Side=Right
  B+ : PMIOPort  Port=3  Side=Left
  B- : PMIOPort  Port=4  Side=Right
  C+ : PMIOPort  Port=5  Side=Left
  C- : PMIOPort  Port=6  Side=Right
  connections:
  Lgc/RConn1 -- Cfc/LConn1 -- Lic/LConn1
  Lgb/RConn1 -- Cfb/LConn1 -- Lib/LConn1
  Lgc/LConn1 -- C+/RConn1
  Cfa/RConn1 -- Rda/LConn1
  Lgb/LConn1 -- B+/RConn1
  Lic/RConn1 -- C-/RConn1
  Lia/LConn1 -- Cfa/LConn1 -- Lga/RConn1
  Lib/RConn1 -- B-/RConn1
  Lia/RConn1 -- A-/RConn1
  Lga/LConn1 -- A+/RConn1
  Rda/RConn1 -- " Rdb"/RConn1 -- Rdc/RConn1
  Cfb/RConn1 -- " Rdb"/LConn1
  Rdc/LConn1 -- Cfc/RConn1

== system three_phase_bidirectional_EV_charger_simscape/          /             ==
  a : Inport
  b : Inport  Port=2
  c : Inport  Port=3
  theta : Inport  Port=4
  abc to dqs (stationary) : Subsystem
  dqs to dqe (rotating) : Subsystem
  d : Outport
  q : Outport  Port=2
  wires:
  abc to dqs (stationary)/1(qs) -> dqs to dqe (rotating)/1("qs ")
  dqs to dqe (rotating)/2("qe ") -> q/1
  abc to dqs (stationary)/2(ds) -> dqs to dqe (rotating)/2("ds ")
  a/1 -> abc to dqs (stationary)/1(a)
  b/1 -> abc to dqs (stationary)/2(b)
  c/1 -> abc to dqs (stationary)/3(c)
  dqs to dqe (rotating)/1("de ") -> d/1
  theta/1 -> dqs to dqe (rotating)/3(theta)

== system three_phase_bidirectional_EV_charger_simscape/          /                     ==
  a : Inport
  b : Inport  Port=2
  c : Inport  Port=3
  theta : Inport  Port=4
  abc to dqs (stationary) : Subsystem
  dqs to dqe (rotating) : Subsystem
  d : Outport
  q : Outport  Port=2
  wires:
  abc to dqs (stationary)/1(qs) -> dqs to dqe (rotating)/1("qs ")
  dqs to dqe (rotating)/2("qe ") -> q/1
  abc to dqs (stationary)/2(ds) -> dqs to dqe (rotating)/2("ds ")
  a/1 -> abc to dqs (stationary)/1(a)
  b/1 -> abc to dqs (stationary)/2(b)
  c/1 -> abc to dqs (stationary)/3(c)
  dqs to dqe (rotating)/1("de ") -> d/1
  theta/1 -> dqs to dqe (rotating)/3(theta)

== system three_phase_bidirectional_EV_charger_simscape/          /                                                                                                                                                                                                                                                    ==
  note: Inverse Clark-Park Transformation
  q : Inport
  d : Inport  Port=2
  theta : Inport  Port=3
  dqe to dqs : Subsystem
  dqs to abc : Subsystem
  a : Outport
  b : Outport  Port=2
  c : Outport  Port=3
  wires:
  d/1 -> dqe to dqs/2("de ")
  dqe to dqs/1("qs ") -> dqs to abc/1(qs)
  q/1 -> dqe to dqs/1("qe ")
  dqe to dqs/2(ds) -> dqs to abc/2(ds)
  dqs to abc/3(c) -> c/1
  dqs to abc/2(b) -> b/1
  dqs to abc/1(a) -> a/1
  theta/1 -> dqe to dqs/3(theta)

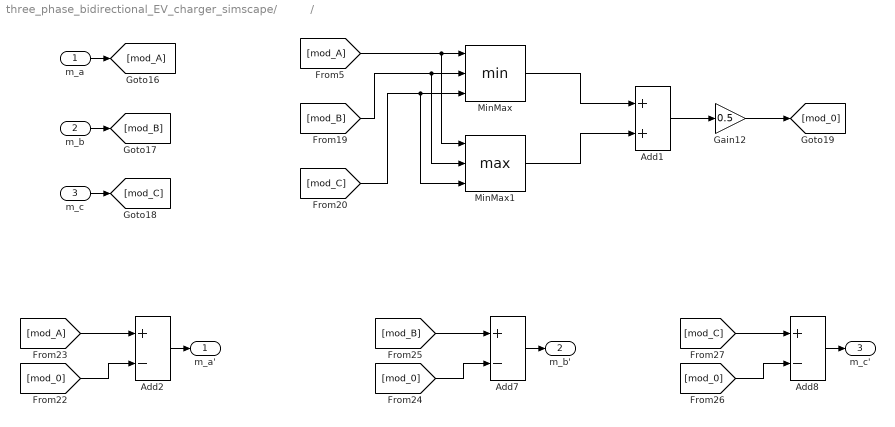
== system three_phase_bidirectional_EV_charger_simscape/          /                                                                                                                                                                                                                                                               ==
  m_a : Inport
  m_b : Inport  Port=2
  m_c : Inport  Port=3
  Add1 : Sum
  Add2 : Sum  Inputs=+-
  Add7 : Sum  Inputs=+-
  Add8 : Sum  Inputs=+-
  Gain12 : Gain  Gain=0.5
  MinMax : MinMax  Inputs=3
  MinMax1 : MinMax  Function=max  Inputs=3
  m_a' : Outport
  m_b' : Outport  Port=2
  m_c' : Outport  Port=3
  wires:
  [mod_0] -> Add8/2
  Gain12/1 -> [mod_0]
  MinMax1/1 -> Add1/2
  [mod_C] -> MinMax1/3, MinMax/3
  [mod_A] -> Add2/1
  [mod_0] -> Add2/2
  [mod_C] -> Add8/1
  m_b/1 -> [mod_B]
  Add8/1 -> m_c'/1
  [mod_A] -> MinMax1/1, MinMax/1
  [mod_0] -> Add7/2
  [mod_B] -> Add7/1
  [mod_B] -> MinMax1/2, MinMax/2
  Add1/1 -> Gain12/1
  MinMax/1 -> Add1/1
  m_a/1 -> [mod_A]
  Add2/1 -> m_a'/1
  m_c/1 -> [mod_C]
  Add7/1 -> m_b'/1

== system three_phase_bidirectional_EV_charger_simscape/          /DC link variation g2v ==
  Add : Sum
  Step : Step  Time=0.075  After=1.2  SampleTime=0
  Step1 : Step  Time=0.09  After=-1.2  SampleTime=0
  Vbus_step : Outport
  wires:
  Add/1 -> Vbus_step/1
  Step/1 -> Add/1
  Step1/1 -> Add/2
